simulink model "parallel_three_phase_converter"  (R2022b)
settings: Solver=VariableStepAuto  StartTime=0.0  StopTime=2  FixedStep=1e-6  MaxStep=1e-7  RelTol=1e-5
model workspace (MAT data in the model file):
  wr = 314.159265359
undefined symbols (not defined in the file): DiscIntNeverNeededParam, Ts
libraries: spsMosfetLib x12, spsCurrentMeasurementLib x7, dspsigops x7, slpidlib x5, simulink x3, spsThreePhaseSeriesRLCBranchLib x3, spsVoltageMeasurementLib x3, spsDCVoltageSourceLib x1, spsThreePhaseBreakerLib x1, spspowerguiLib x1
settings Model: Creator=SSC  LastModifiedBy=SSC

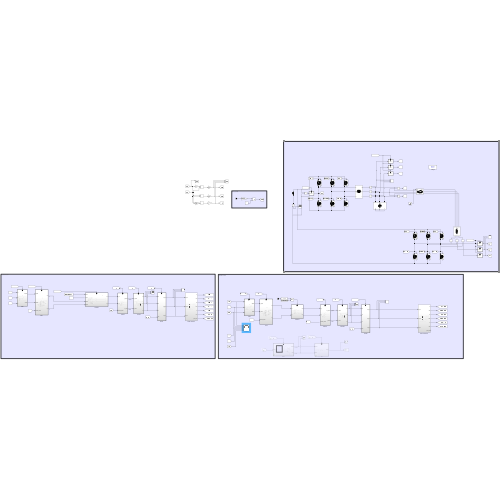
[thumbnail: Simulink's stored preview of the top-level diagram]
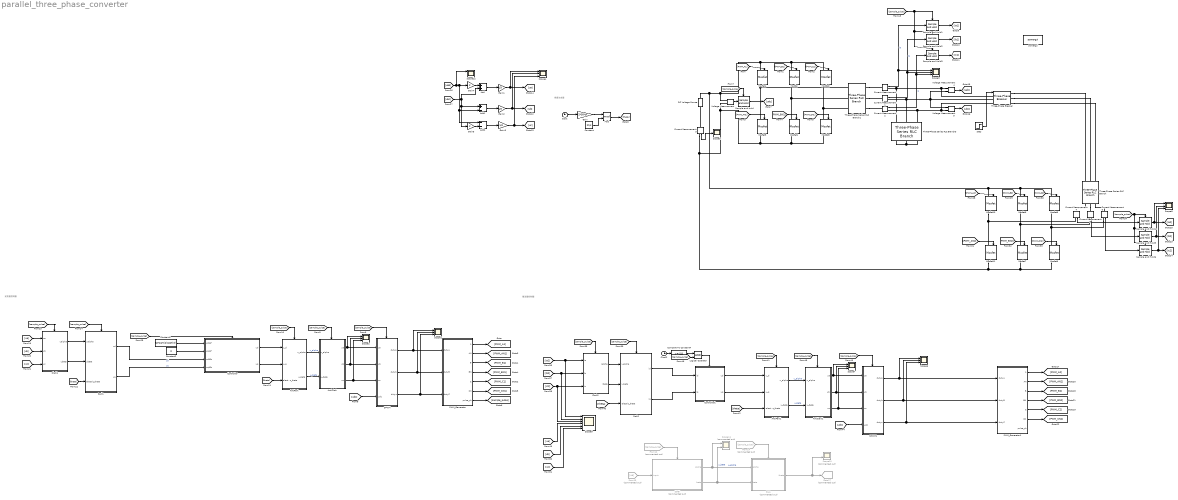
== system parallel_three_phase_converter ==
  note: 角度生成器
  note: 逆变器控制器
  note: 整流器控制器
  Add : Sum
  Add1 : Sum  Inputs=+-
  Add2 : Sum  Inputs=--
  AntiClark : Subsystem
  AntiClark1 : Subsystem
  AntiPark : Subsystem
  AntiPark1 : Subsystem
  Clark1 : Subsystem
  Clark2 : Subsystem
  Clock : Clock
  Clock2 : Clock
  Compare To Constant4 : simulink/Logic and Bit Operations/Compare To Constant  relop=>=  const=0.8  OutDataTypeStr=boolean
  Constant : Constant  Value=2*pi
  Constant1 : Constant  Value=32*sqrt(2)/sqrt(3)
  Constant2 : Constant  Value=0
  Controller : Subsystem
  Controller1 : Subsystem
  Current Measurement{,1..6} (7 alike) : spsCurrentMeasurementLib/Current Measurement  PhasorSimulation=off  OutputType=Complex  PSBequivalent=0
  DC Voltage Source : spsDCVoltageSourceLib/DC Voltage Source  Amplitude=56  Measurements=None
  From12 : From  Commented=on  GotoTag=sample_pulse
  From13 : From  Commented=on  GotoTag=ua
  From14 : From  Commented=on  GotoTag=sample_pulse
  Gain : Gain  Gain=2*50*pi
  Gain1 : Gain  Gain=1/3
  Gain2 : Gain  Gain=1/3
  Gain3 : Gain  Gain=1/3
  Gain4 : Gain  Gain=2
  Gain5 : Gain  Gain=2
  Goto27 : Goto  Commented=on  GotoTag=us_theta
  Logical Operator : Logic  AllPortsSameDT=off  OutDataTypeStr=boolean
  Mod : Math  Operator=mod
  Mosfet{,1..11} (12 alike) : spsMosfetLib/Mosfet  Ron=0.1  Lon=0  Rd=0.01  Vfd=0  IC=0  Rs=1e5  Cs=inf  Measurements=on
  PLL1 : Subsystem  Commented=on  TreatAsAtomicUnit=on
  PWM_Generator : Subsystem
  PWM_Generator1 : Subsystem
  Park1 : Subsystem
  Park2 : Subsystem
  SOGI : Subsystem  Commented=on  TreatAsAtomicUnit=on
  SPWM : Subsystem
  SPWM1 : Subsystem
  Sample and Hold{,1..6} (7 alike) : dspsigops/Sample and Hold  trig=Rising edge  initCond=0  latchinput=off
  Scope{1..4,6..8,12} (8 alike) : Scope  NumInputPorts=3
  Scope10 : Scope  Commented=on  NumInputPorts=2
  Scope11 : Scope  Commented=on  NumInputPorts=2
  Scope5 : Scope
  Scope9 : Scope  NumInputPorts=6
  Step : Step  Time=0.8  SampleTime=0
  Three-Phase Series RLC Branch : spsThreePhaseSeriesRLCBranchLib/Three-Phase Series RLC Branch  LConnTagsString=A|B|C  RConnTagsString=A|B|C  BranchType=L  Resistance=0  Inductance=2e-3  Capacitance=1e-6  Measurements=None
  Three-Phase Series RLC Branch1 : spsThreePhaseSeriesRLCBranchLib/Three-Phase Series RLC Branch  LConnTagsString=A|B|C  RConnTagsString=A|B|C  BranchType=L  Resistance=0  Inductance=2e-3  Capacitance=1e-6  Measurements=None
  Three-Phase Series RLC Branch3 : spsThreePhaseSeriesRLCBranchLib/Three-Phase Series RLC Branch  LConnTagsString=A|B|C  RConnTagsString=A|B|C  BranchType=C  Resistance=0  Inductance=10e-3  Capacitance=25e-6  Measurements=None
  Three-Phase Breaker : spsThreePhaseBreakerLib/Three-Phase Breaker  InitialState=open  SwitchA=on  SwitchB=on  SwitchC=on  SwitchTimes="[1/60  5/60]"  External=on  BreakerResistance=0.01  SnubberResistance=1e6  SnubberCapacitance=inf  Measurements=None
  Voltage Measurement : spsVoltageMeasurementLib/Voltage Measurement  PhasorSimulation=off  OutputType=Complex  PSBequivalent=0
  Voltage Measurement4 : spsVoltageMeasurementLib/Voltage Measurement  PhasorSimulation=off  OutputType=Complex  PSBequivalent=0
  Voltage Measurement5 : spsVoltageMeasurementLib/Voltage Measurement  PhasorSimulation=off  OutputType=Complex  PSBequivalent=0
  powergui : spspowerguiLib/powergui  Priority=1  SimulationMode=Discrete  SampleTime=1e-7  frequency=60  Iterations=50  frequencyindice=0  Pbase=100e6  ErrMax=1e-4  UnitsV=kV  UnitsW=MW  buscounter=0  FunctionMessages=off  echomessages=off  EnableUseOfTLC=off  CurrentSourceSwitches=off  DisableSnubberDevices=off  DisableRonSwitches=off  DisableVfSwitches=off  DisplayEquations=off  AutomaticDiscreteSolvers=off  SolverType=Tustin/Backward Euler (TBE)  Interpol=off  ExternalGateDelay=off  methode=off  Ts=100  x0status=blocks  SPID=on  SwTol=0  HookPort=off  NonlinearTolerance=1e-4  nMaxIteration=100  ContinueOnMaxIteration=off  RestoreLinks=warning  ResistiveCurrentMeasurement=off  Frange=[0:2:500]  Ylog=off  Xlog=on  ShowGrid=off  save=off  variable=ZData  structure=0  ZoomFFT=off  StartTime=0.0  cycles=1  DisplayStyle=1  fundamental=60  FreqAxis=off  MaxFrequency=1000  frequencyindicesteady=1  RmsSteady=1  display=off
  wires:
  Add/1 -> Gain1/1
  [uab] -> Scope12/1, Gain4/1, Add2/1, Add1/2
  Voltage Measurement5/1 -> [ubc]
  Add2/1 -> Gain3/1
  Voltage Measurement4/1 -> [uab]
  [ubc] -> Add/2, Gain5/1, Add1/1
  Gain3/1 -> Scope4/3, [uc]
  [ub] -> Clark1/2(ub)
  [theta] -> Park1/3(electric_theta)
  Park1/2(uq) -> Controller/4(uqfdb)  "uq"
  Clark1/2(ubeta) -> Park1/2(ubeta)
  [sample_pulse] -> Sample and Hold/Trigger
  Controller/2(uq) -> AntiPark/2(u_q)
  [sample_pulse] -> Park1/Trigger
  [PWM_A1] -> Mosfet4/1
  Constant2/1 -> Controller/2(uqref)
  Constant1/1 -> Controller/1(udref)
  Sample and Hold3/1 -> [ic1]
  [sample_pulse] -> Clark1/Trigger
  PWM_Generator/3(B) -> [PWM_B1]
  Sample and Hold1/1 -> [ia1]
  Current Measurement1/1 -> Scope3/2, Sample and Hold2/1  "ib"
  AntiClark/2(ub) -> SPWM/2(ub), Scope2/2
  SPWM/1(dutya) -> Scope1/1, PWM_Generator/1(dutyA)
  SPWM/2(dutyb) -> Scope1/2, PWM_Generator/2(dutyB)
  [sample_pulse] -> Controller/Trigger
  Sample and Hold/1 -> [udc]
  [ua] -> Clark1/1(ua)
  [udc] -> SPWM/4(udc)
  Controller/1(ud) -> AntiPark/1(u_d)
  [sample_pulse] -> AntiPark/Trigger
  Sample and Hold2/1 -> [ib1]
  Constant/1 -> Mod/2
  AntiClark/3(uc) -> SPWM/3(uc), Scope2/3
  Current Measurement2/1 -> Scope3/3, Sample and Hold3/1  "ic"
  [PWM_BN1] -> Mosfet1/1
  [PWM_B1] -> Mosfet/1
  PWM_Generator/6(CN) -> [PWM_CN1]
  Current Measurement/1 -> Scope3/1, Sample and Hold1/1  "ia"
  PWM_Generator/2(AN) -> [PWM_AN1]
  PWM_Generator/4(BN) -> [PWM_BN1]
  [sample_pulse] -> AntiClark/Trigger
  Voltage Measurement/1 -> Sample and Hold/1
  PWM_Generator/1(A) -> [PWM_A1]
  [PWM_AN1] -> Mosfet5/1
  [sample_pulse] -> SPWM/Trigger
  PWM_Generator/7(pulse_sh) -> [sample_pulse]
  SPWM/3(dutyc) -> Scope1/3, PWM_Generator/3(dutyC)
  [PWM_CN1] -> Mosfet3/1
  Clock/1 -> Gain/1
  [uc] -> Clark1/3(uc)
  AntiClark/1(ua) -> SPWM/1(ua), Scope2/1
  Gain5/1 -> Add2/2
  Gain/1 -> Mod/1
  Gain4/1 -> Add/1
  PWM_Generator/5(C) -> [PWM_C1]
  [PWM_C1] -> Mosfet2/1
  Gain2/1 -> Scope4/2, [ub]
  Mod/1 -> [theta]
  [theta] -> AntiPark/3(electric_theta)
  Add1/1 -> Gain2/1
  [sample_pulse] -> Sample and Hold1/Trigger, Sample and Hold3/Trigger, Sample and Hold2/Trigger
  [PWM_C2] -> Mosfet8/1
  [PWM_CN2] -> Mosfet9/1
  [PWM_AN2] -> Mosfet11/1
  [PWM_BN2] -> Mosfet7/1
  [PWM_B2] -> Mosfet6/1
  [PWM_A2] -> Mosfet10/1
  SPWM1/1(dutya) -> PWM_Generator1/1(dutyA), Scope6/1
  SPWM1/2(dutyb) -> PWM_Generator1/2(dutyB), Scope6/2
  SPWM1/3(dutyc) -> PWM_Generator1/3(dutyC), Scope6/3
  Current Measurement3/1 -> Scope5/1
  Current Measurement5/1 -> Sample and Hold5/1
  Current Measurement4/1 -> Sample and Hold4/1
  Current Measurement6/1 -> Sample and Hold6/1
  [sample_pulse] -> Sample and Hold4/Trigger, Sample and Hold6/Trigger, Sample and Hold5/Trigger
  Clark2/2(ibeta) -> Park2/2(i_beta)
  [sample_pulse] -> Park2/Trigger
  [ib2] -> Scope9/2, Clark2/2(ib)
  [ia2] -> Scope9/1, Clark2/1(ia)
  [sample_pulse] -> Clark2/Trigger
  Clark2/1(ialpha) -> Park2/1(i_alpha)
  AntiClark1/1(ua) -> SPWM1/1(ua), Scope7/1
  [sample_pulse] -> AntiClark1/Trigger
  [sample_pulse] -> SPWM1/Trigger
  AntiPark1/1(u_alpha) -> AntiClark1/1(u_alpha)  "u_alpha"
  [sample_pulse] -> AntiPark1/Trigger
  AntiClark1/3(uc) -> SPWM1/3(uc), Scope7/3
  [udc] -> SPWM1/4(udc)
  AntiClark1/2(ub) -> SPWM1/2(ub), Scope7/2
  AntiPark1/2(u_beta) -> AntiClark1/2(u_beta)  "u_beta"
  Park2/1(id) -> Controller1/1(id)
  Park2/2(iq) -> Controller1/2(iq)
  PWM_Generator1/1(A) -> [PWM_A2]
  PWM_Generator1/2(AN) -> [PWM_AN2]
  PWM_Generator1/4(BN) -> [PWM_BN2]
  PWM_Generator1/3(B) -> [PWM_B2]
  PWM_Generator1/5(C) -> [PWM_C2]
  PWM_Generator1/6(CN) -> [PWM_CN2]
  Controller1/1(ud) -> AntiPark1/1(u_d)
  Controller1/2(uq) -> AntiPark1/2(u_q)
  AntiPark/1(u_alpha) -> AntiClark/1(u_alpha)  "u_alpha"
  AntiPark/2(u_beta) -> AntiClark/2(u_beta)  "u_beta"
  Gain1/1 -> Scope4/1, [ua]
  Clark1/1(ualpha) -> Park1/1(ualpha)
  [theta] -> AntiPark1/3(electric_theta)
  Park1/1(ud) -> Controller/3(udfdb)  "ud"
  [ua] -> Scope9/4
  [uc] -> Scope9/6
  Sample and Hold4/1 -> Scope8/1, [ia2]
  Sample and Hold5/1 -> Scope8/2, [ib2]
  Sample and Hold6/1 -> Scope8/3, [ic2]
  [theta] -> Park2/3(electric_theta)
  [ub] -> Scope9/5
  Clock2/1 -> Compare To Constant4/1
  Compare To Constant4/1 -> Logical Operator/1
  [sample_pulse] -> Logical Operator/2
  Logical Operator/1 -> Controller1/Trigger
  [ic2] -> Scope9/3, Clark2/3(ic)
  SOGI/1(alpha) -> PLL1/1(alpha), Scope11/1  "u_alpha"
  From12/1 -> SOGI/Trigger
  SOGI/2(beta) -> PLL1/2(beta), Scope11/2  "u_beta"
  From13/1 -> SOGI/1(input)
  From14/1 -> PLL1/Trigger
  PLL1/1(theta) -> Scope10/2, Goto27/1
  Step/1 -> Three-Phase Breaker/1
  connections:
  Mosfet11/RConn1 -- Mosfet1/RConn1 -- Mosfet3/RConn1 -- Mosfet5/RConn1 -- Voltage Measurement/LConn2 -- Current Measurement3/RConn1 -- Mosfet9/RConn1 -- Mosfet7/RConn1
  Mosfet8/LConn1 -- Mosfet6/LConn1 -- Mosfet4/LConn1 -- Mosfet/LConn1 -- Mosfet2/LConn1 -- Voltage Measurement/LConn1 -- DC Voltage Source/RConn1 -- Mosfet10/LConn1
  Mosfet/RConn1 -- Three-Phase Series RLC Branch1/LConn2 -- Mosfet1/LConn1
  Mosfet4/RConn1 -- Three-Phase Series RLC Branch1/LConn1 -- Mosfet5/LConn1
  Mosfet2/RConn1 -- Three-Phase Series RLC Branch1/LConn3 -- Mosfet3/LConn1
  Three-Phase Series RLC Branch1/RConn1 -- Current Measurement/LConn1
  Three-Phase Series RLC Branch1/RConn2 -- Current Measurement1/LConn1
  Three-Phase Series RLC Branch1/RConn3 -- Current Measurement2/LConn1
  Mosfet9/LConn1 -- Current Measurement6/RConn1 -- Mosfet8/RConn1
  Mosfet10/RConn1 -- Current Measurement4/RConn1 -- Mosfet11/LConn1
  Mosfet7/LConn1 -- Current Measurement5/RConn1 -- Mosfet6/RConn1
  Current Measurement/RConn1 -- Three-Phase Breaker/LConn1 -- Voltage Measurement4/LConn1 -- Three-Phase Series RLC Branch3/LConn1
  Current Measurement1/RConn1 -- Three-Phase Breaker/LConn2 -- Voltage Measurement5/LConn1 -- Voltage Measurement4/LConn2 -- Three-Phase Series RLC Branch3/LConn2
  Current Measurement2/RConn1 -- Three-Phase Breaker/LConn3 -- Voltage Measurement5/LConn2 -- Three-Phase Series RLC Branch3/LConn3
  Three-Phase Series RLC Branch/RConn1 -- Current Measurement4/LConn1
  Three-Phase Series RLC Branch/RConn2 -- Current Measurement5/LConn1
  Three-Phase Series RLC Branch/RConn3 -- Current Measurement6/LConn1
  Current Measurement3/LConn1 -- DC Voltage Source/LConn1
  Three-Phase Series RLC Branch3/RConn1 -- Three-Phase Series RLC Branch3/RConn3 -- Three-Phase Series RLC Branch3/RConn2
  Three-Phase Breaker/RConn3 -- Three-Phase Series RLC Branch/LConn3
  Three-Phase Breaker/RConn2 -- Three-Phase Series RLC Branch/LConn2
  Three-Phase Breaker/RConn1 -- Three-Phase Series RLC Branch/LConn1

== system parallel_three_phase_converter/AntiClark ==
  u_alpha : Inport
  u_beta : Inport  Port=2
  Trigger : TriggerPort  VariantControl=(inherit)
  Gain : Gain  Gain=-1/2
  Gain1 : Gain  Gain=sqrt(3)/2
  Sum : Sum  Inputs=|++
  Sum1 : Sum  Inputs=-+|
  ua : Outport
  ub : Outport  Port=2
  uc : Outport  Port=3
  wires:
  Sum1/1 -> uc/1
  Gain1/1 -> Sum1/1, Sum/2
  Sum/1 -> ub/1
  Gain/1 -> Sum/1, Sum1/2
  u_beta/1 -> Gain1/1
  u_alpha/1 -> ua/1, Gain/1

== system parallel_three_phase_converter/AntiClark1 ==
  u_alpha : Inport
  u_beta : Inport  Port=2
  Trigger : TriggerPort  VariantControl=(inherit)
  Gain : Gain  Gain=-1/2
  Gain1 : Gain  Gain=sqrt(3)/2
  Sum : Sum  Inputs=|++
  Sum1 : Sum  Inputs=-+|
  ua : Outport
  ub : Outport  Port=2
  uc : Outport  Port=3
  wires:
  Sum1/1 -> uc/1
  Gain1/1 -> Sum1/1, Sum/2
  Sum/1 -> ub/1
  Gain/1 -> Sum/1, Sum1/2
  u_beta/1 -> Gain1/1
  u_alpha/1 -> ua/1, Gain/1

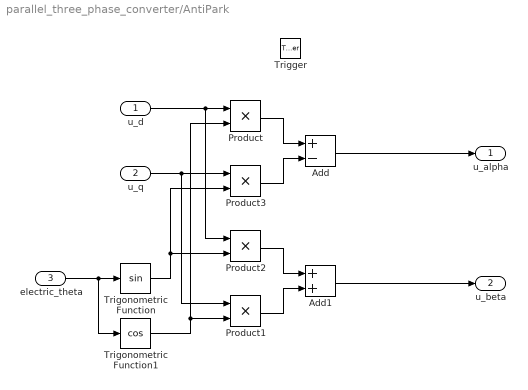
== system parallel_three_phase_converter/AntiPark ==
  u_d : Inport
  u_q : Inport  Port=2
  electric_theta : Inport  Port=3
  Trigger : TriggerPort  VariantControl=(inherit)
  Add : Sum  Inputs=+-
  Add1 : Sum
  Product{,1..3} (4 alike) : Product
  Trigonometric Function : Trigonometry
  Trigonometric Function1 : Trigonometry  Operator=cos
  u_alpha : Outport
  u_beta : Outport  Port=2
  wires:
  electric_theta/1 -> Trigonometric Function1/1, Trigonometric Function/1
  u_d/1 -> Product2/1, Product/1
  Trigonometric Function1/1 -> Product/2, Product1/2
  u_q/1 -> Product1/1, Product3/1
  Trigonometric Function/1 -> Product2/2, Product3/2
  Product/1 -> Add/1
  Product3/1 -> Add/2
  Add/1 -> u_alpha/1
  Product2/1 -> Add1/1
  Product1/1 -> Add1/2
  Add1/1 -> u_beta/1

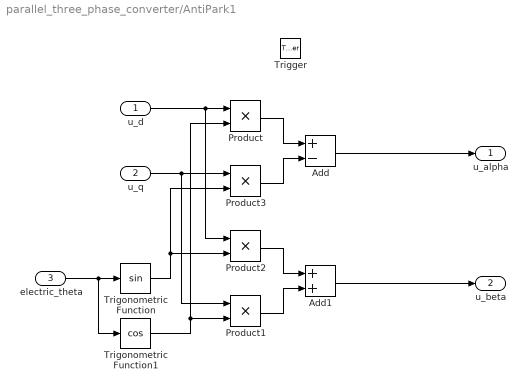
== system parallel_three_phase_converter/AntiPark1 ==
  u_d : Inport
  u_q : Inport  Port=2
  electric_theta : Inport  Port=3
  Trigger : TriggerPort  VariantControl=(inherit)
  Add : Sum  Inputs=+-
  Add1 : Sum
  Product{,1..3} (4 alike) : Product
  Trigonometric Function : Trigonometry
  Trigonometric Function1 : Trigonometry  Operator=cos
  u_alpha : Outport
  u_beta : Outport  Port=2
  wires:
  electric_theta/1 -> Trigonometric Function1/1, Trigonometric Function/1
  u_d/1 -> Product2/1, Product/1
  Trigonometric Function1/1 -> Product/2, Product1/2
  u_q/1 -> Product1/1, Product3/1
  Trigonometric Function/1 -> Product2/2, Product3/2
  Product/1 -> Add/1
  Product3/1 -> Add/2
  Add/1 -> u_alpha/1
  Product2/1 -> Add1/1
  Product1/1 -> Add1/2
  Add1/1 -> u_beta/1

== system parallel_three_phase_converter/Clark1 ==
  ua : Inport
  ub : Inport  Port=2
  uc : Inport  Port=3
  Trigger : TriggerPort  VariantControl=(inherit)
  Add : Sum
  Add1 : Sum  Inputs=+-
  Add2 : Sum  Inputs=+-
  Gain : Gain  Gain=2/3
  Gain1 : Gain  Gain=1/3
  Gain2 : Gain  Gain=sqrt(3)/3
  ualpha : Outport
  ubeta : Outport  Port=2
  wires:
  ua/1 -> Gain/1
  ub/1 -> Add1/1, Add/1
  uc/1 -> Add/2, Add1/2
  Add/1 -> Gain1/1
  Add1/1 -> Gain2/1
  Gain/1 -> Add2/1
  Gain1/1 -> Add2/2
  Add2/1 -> ualpha/1
  Gain2/1 -> ubeta/1

== system parallel_three_phase_converter/Clark2 ==
  ia : Inport
  ib : Inport  Port=2
  ic : Inport  Port=3
  Trigger : TriggerPort  VariantControl=(inherit)
  Add : Sum
  Add1 : Sum  Inputs=+-
  Add2 : Sum  Inputs=+-
  Gain : Gain  Gain=2/3
  Gain1 : Gain  Gain=1/3
  Gain2 : Gain  Gain=sqrt(3)/3
  ialpha : Outport
  ibeta : Outport  Port=2
  wires:
  ia/1 -> Gain/1
  ib/1 -> Add1/1, Add/1
  ic/1 -> Add/2, Add1/2
  Add/1 -> Gain1/1
  Add1/1 -> Gain2/1
  Gain/1 -> Add2/1
  Gain1/1 -> Add2/2
  Add2/1 -> ialpha/1
  Gain2/1 -> ibeta/1

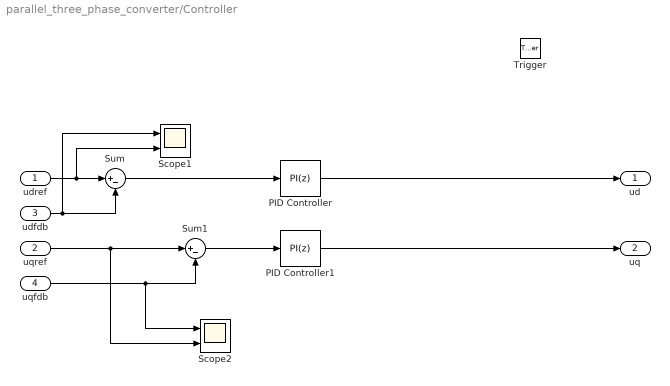
== system parallel_three_phase_converter/Controller ==
  udref : Inport
  uqref : Inport  Port=2
  udfdb : Inport  Port=3
  uqfdb : Inport  Port=4
  Trigger : TriggerPort  VariantControl=(inherit)
  PID Controller : slpidlib/PID Controller  Controller=PI  Form=Parallel  TimeDomain=Discrete-time  UseExternalTs=off  SampleTime=-1  IntegratorMethod=Forward Euler  FilterMethod=Forward Euler  ControllerParametersSource=internal  P=0.01  I=5  UseKiTs=off  D=0  N=100  UseFilter=on  TunerSelectOption=Transfer Function Based (PID Tuner App)  InitialConditionSource=internal  InitialConditionForIntegrator=0  InitialConditionForFilter=0  DifferentiatorICPrevScaledInput=0  ExternalReset=none  TrackingMode=off  Kt=1  LimitOutput=on  SatLimitsSource=internal  UpperSaturationLimit=60/2  LowerSaturationLimit=-60/2  LinearizeAsGain=on  AntiWindupMode=clamping  Kb=1  LimitIntegrator=off  UpperIntegratorSaturationLimit=inf  LowerIntegratorSaturationLimit=-inf  POutMin=[]  POutMax=[]  IOutMin=[]  IOutMax=[]  DOutMin=[]  DOutMax=[]  NOutMin=[]  NOutMax=[]  SumOutMin=[]  SumOutMax=[]  SaturationOutMin=[]  SaturationOutMax=[]  PParamMin=[]  PParamMax=[]  IParamMin=[]  IParamMax=[]  DParamMin=[]  DParamMax=[]  NParamMin=[]  NParamMax=[]  KbParamMin=[]  KbParamMax=[]  KtParamMin=[]  KtParamMax=[]  KbOutMin=[]  KbOutMax=[]  KtOutMin=[]  KtOutMax=[]  IntegratorOutMin=[]  IntegratorOutMax=[]  FilterOutMin=[]  FilterOutMax=[]  SumI1OutMin=[]  SumI1OutMax=[]  SumI2OutMin=[]  SumI2OutMax=[]  SumI3OutMin=[]  SumI3OutMax=[]  SumI4OutMin=[]  SumI4OutMax=[]  SumDOutMin=[]  SumDOutMax=[]  DifferentiatorOutMin=[]  DifferentiatorOutMax=[]  FilterDiffOutCoefMin=[]  FilterDiffOutCoefMax=[]  ReciprocalOutMin=[]  ReciprocalOutMax=[]  SumDenOutMin=[]  SumDenOutMax=[]  SumNumOutMin=[]  SumNumOutMax=[]  DivideOutMin=[]  DivideOutMax=[]  UdiffTsProdOutMin=[]  UdiffTsProdOutMax=[]  NTsProdOutMin=[]  NTsProdOutMax=[]  UintegralTsProdOutMin=[]  UintegralTsProdOutMax=[]  UngainTsProdOutMin=[]  UngainTsProdOutMax=[]  ClampingZeroOutDataTypeStr=Inherit: Inherit via back propagation  ClampingZeroOutMin=[]  ClampingZeroOutMax=[]  FilterDenConstantOutDataTypeStr=Inherit: Inherit via back propagation  FilterDenConstantOutMin=[]  FilterDenConstantOutMax=[]  PCopyOutDataTypeStr=Inherit: Inherit via back propagation  PCopyOutMin=[]  PCopyOutMax=[]  NCopyOutDataTypeStr=Inherit: Inherit via back propagation  NCopyOutMin=[]  NCopyOutMax=[]  IntegratorContinuousStateAttributes=''  IntegratorStateMustResolveToSignalObject=off  IntegratorRTWStateStorageClass=Auto  FilterContinuousStateAttributes=''  FilterStateMustResolveToSignalObject=off  FilterRTWStateStorageClass=Auto  ParallelPVariant=InternalParameters  IdealPVariant=Disabled  IVariant=InternalParameters  DVariant=Disabled  IntegratorVariant=Discrete  SatVariant=Enabled  AWVariant=DiscClampingParallel  PCopyVariant=Disabled  TRVariant=Disabled  FdbkBlocksVariant=Forward  IdealPFdbkVariant=Disabled  SatFdbkVariant=Disabled  DerivativeFilterVariant=Disabled  NVariant=Disabled  NCopyVariant=Disabled_SignalSpec  FilterICVariant=Disabled  IntegratorICVariant=InternalICs  ExternalResetVariant=Disabled  TRSumVariant=Passthrough  SumFdbkVariant=Disabled  SumVariant=Sum_PI  TsampFilterVariant=InternalTs  TsampNgainVariant=Passthrough  TsampIntegralVariant=Passthrough  ExternalSaturationOutDataTypeStr=Inherit: Same as second input
  PID Controller1 : slpidlib/PID Controller  Controller=PI  Form=Parallel  TimeDomain=Discrete-time  UseExternalTs=off  SampleTime=-1  IntegratorMethod=Forward Euler  FilterMethod=Forward Euler  ControllerParametersSource=internal  P=0.01  I=5  UseKiTs=off  D=0  N=100  UseFilter=on  TunerSelectOption=Transfer Function Based (PID Tuner App)  InitialConditionSource=internal  InitialConditionForIntegrator=0  InitialConditionForFilter=0  DifferentiatorICPrevScaledInput=0  ExternalReset=none  TrackingMode=off  Kt=1  LimitOutput=on  SatLimitsSource=internal  UpperSaturationLimit=60/2  LowerSaturationLimit=-60/2  LinearizeAsGain=on  AntiWindupMode=clamping  Kb=1  LimitIntegrator=off  UpperIntegratorSaturationLimit=inf  LowerIntegratorSaturationLimit=-inf  POutMin=[]  POutMax=[]  IOutMin=[]  IOutMax=[]  DOutMin=[]  DOutMax=[]  NOutMin=[]  NOutMax=[]  SumOutMin=[]  SumOutMax=[]  SaturationOutMin=[]  SaturationOutMax=[]  PParamMin=[]  PParamMax=[]  IParamMin=[]  IParamMax=[]  DParamMin=[]  DParamMax=[]  NParamMin=[]  NParamMax=[]  KbParamMin=[]  KbParamMax=[]  KtParamMin=[]  KtParamMax=[]  KbOutMin=[]  KbOutMax=[]  KtOutMin=[]  KtOutMax=[]  IntegratorOutMin=[]  IntegratorOutMax=[]  FilterOutMin=[]  FilterOutMax=[]  SumI1OutMin=[]  SumI1OutMax=[]  SumI2OutMin=[]  SumI2OutMax=[]  SumI3OutMin=[]  SumI3OutMax=[]  SumI4OutMin=[]  SumI4OutMax=[]  SumDOutMin=[]  SumDOutMax=[]  DifferentiatorOutMin=[]  DifferentiatorOutMax=[]  FilterDiffOutCoefMin=[]  FilterDiffOutCoefMax=[]  ReciprocalOutMin=[]  ReciprocalOutMax=[]  SumDenOutMin=[]  SumDenOutMax=[]  SumNumOutMin=[]  SumNumOutMax=[]  DivideOutMin=[]  DivideOutMax=[]  UdiffTsProdOutMin=[]  UdiffTsProdOutMax=[]  NTsProdOutMin=[]  NTsProdOutMax=[]  UintegralTsProdOutMin=[]  UintegralTsProdOutMax=[]  UngainTsProdOutMin=[]  UngainTsProdOutMax=[]  ClampingZeroOutDataTypeStr=Inherit: Inherit via back propagation  ClampingZeroOutMin=[]  ClampingZeroOutMax=[]  FilterDenConstantOutDataTypeStr=Inherit: Inherit via back propagation  FilterDenConstantOutMin=[]  FilterDenConstantOutMax=[]  PCopyOutDataTypeStr=Inherit: Inherit via back propagation  PCopyOutMin=[]  PCopyOutMax=[]  NCopyOutDataTypeStr=Inherit: Inherit via back propagation  NCopyOutMin=[]  NCopyOutMax=[]  IntegratorContinuousStateAttributes=''  IntegratorStateMustResolveToSignalObject=off  IntegratorRTWStateStorageClass=Auto  FilterContinuousStateAttributes=''  FilterStateMustResolveToSignalObject=off  FilterRTWStateStorageClass=Auto  ParallelPVariant=InternalParameters  IdealPVariant=Disabled  IVariant=InternalParameters  DVariant=Disabled  IntegratorVariant=Discrete  SatVariant=Enabled  AWVariant=DiscClampingParallel  PCopyVariant=Disabled  TRVariant=Disabled  FdbkBlocksVariant=Forward  IdealPFdbkVariant=Disabled  SatFdbkVariant=Disabled  DerivativeFilterVariant=Disabled  NVariant=Disabled  NCopyVariant=Disabled_SignalSpec  FilterICVariant=Disabled  IntegratorICVariant=InternalICs  ExternalResetVariant=Disabled  TRSumVariant=Passthrough  SumFdbkVariant=Disabled  SumVariant=Sum_PI  TsampFilterVariant=InternalTs  TsampNgainVariant=Passthrough  TsampIntegralVariant=Passthrough  ExternalSaturationOutDataTypeStr=Inherit: Same as second input
  Scope1 : Scope  NumInputPorts=2
  Scope2 : Scope  NumInputPorts=2
  Sum : Sum  Inputs=|+-
  Sum1 : Sum  Inputs=|+-
  ud : Outport
  uq : Outport  Port=2
  wires:
  PID Controller1/1 -> uq/1
  uqref/1 -> Scope2/2, Sum1/1
  PID Controller/1 -> ud/1
  udref/1 -> Scope1/2, Sum/1
  Sum/1 -> PID Controller/1
  Sum1/1 -> PID Controller1/1
  udfdb/1 -> Sum/2, Scope1/1
  uqfdb/1 -> Scope2/1, Sum1/2

== system parallel_three_phase_converter/Controller1 ==
  id : Inport
  iq : Inport  Port=2
  Trigger : TriggerPort  VariantControl=(inherit)
  Constant10 : Constant  Value=0
  Constant9 : Constant  Value=0.5
  PID Controller1 : slpidlib/PID Controller  Controller=PI  Form=Parallel  TimeDomain=Discrete-time  UseExternalTs=off  SampleTime=-1  IntegratorMethod=Forward Euler  FilterMethod=Forward Euler  ControllerParametersSource=internal  P=10  I=100  UseKiTs=off  D=0  N=100  UseFilter=on  TunerSelectOption=Transfer Function Based (PID Tuner App)  InitialConditionSource=internal  InitialConditionForIntegrator=0  InitialConditionForFilter=0  DifferentiatorICPrevScaledInput=0  ExternalReset=none  TrackingMode=off  Kt=1  LimitOutput=on  SatLimitsSource=internal  UpperSaturationLimit=60/2  LowerSaturationLimit=-60/2  LinearizeAsGain=on  AntiWindupMode=none  Kb=1  LimitIntegrator=off  UpperIntegratorSaturationLimit=inf  LowerIntegratorSaturationLimit=-inf  POutMin=[]  POutMax=[]  IOutMin=[]  IOutMax=[]  DOutMin=[]  DOutMax=[]  NOutMin=[]  NOutMax=[]  SumOutMin=[]  SumOutMax=[]  SaturationOutMin=[]  SaturationOutMax=[]  PParamMin=[]  PParamMax=[]  IParamMin=[]  IParamMax=[]  DParamMin=[]  DParamMax=[]  NParamMin=[]  NParamMax=[]  KbParamMin=[]  KbParamMax=[]  KtParamMin=[]  KtParamMax=[]  KbOutMin=[]  KbOutMax=[]  KtOutMin=[]  KtOutMax=[]  IntegratorOutMin=[]  IntegratorOutMax=[]  FilterOutMin=[]  FilterOutMax=[]  SumI1OutMin=[]  SumI1OutMax=[]  SumI2OutMin=[]  SumI2OutMax=[]  SumI3OutMin=[]  SumI3OutMax=[]  SumI4OutMin=[]  SumI4OutMax=[]  SumDOutMin=[]  SumDOutMax=[]  DifferentiatorOutMin=[]  DifferentiatorOutMax=[]  FilterDiffOutCoefMin=[]  FilterDiffOutCoefMax=[]  ReciprocalOutMin=[]  ReciprocalOutMax=[]  SumDenOutMin=[]  SumDenOutMax=[]  SumNumOutMin=[]  SumNumOutMax=[]  DivideOutMin=[]  DivideOutMax=[]  UdiffTsProdOutMin=[]  UdiffTsProdOutMax=[]  NTsProdOutMin=[]  NTsProdOutMax=[]  UintegralTsProdOutMin=[]  UintegralTsProdOutMax=[]  UngainTsProdOutMin=[]  UngainTsProdOutMax=[]  ClampingZeroOutDataTypeStr=Inherit: Inherit via back propagation  ClampingZeroOutMin=[]  ClampingZeroOutMax=[]  FilterDenConstantOutDataTypeStr=Inherit: Inherit via back propagation  FilterDenConstantOutMin=[]  FilterDenConstantOutMax=[]  PCopyOutDataTypeStr=Inherit: Inherit via back propagation  PCopyOutMin=[]  PCopyOutMax=[]  NCopyOutDataTypeStr=Inherit: Inherit via back propagation  NCopyOutMin=[]  NCopyOutMax=[]  IntegratorContinuousStateAttributes=''  IntegratorStateMustResolveToSignalObject=off  IntegratorRTWStateStorageClass=Auto  FilterContinuousStateAttributes=''  FilterStateMustResolveToSignalObject=off  FilterRTWStateStorageClass=Auto  ParallelPVariant=InternalParameters  IdealPVariant=Disabled  IVariant=InternalParameters  DVariant=Disabled  IntegratorVariant=Discrete  SatVariant=Enabled  AWVariant=Passthrough  PCopyVariant=Disabled  TRVariant=Disabled  FdbkBlocksVariant=Forward  IdealPFdbkVariant=Disabled  SatFdbkVariant=Disabled  DerivativeFilterVariant=Disabled  NVariant=Disabled  NCopyVariant=Disabled_SignalSpec  FilterICVariant=Disabled  IntegratorICVariant=InternalICs  ExternalResetVariant=Disabled  TRSumVariant=Passthrough  SumFdbkVariant=Disabled  SumVariant=Sum_PI  TsampFilterVariant=InternalTs  TsampNgainVariant=Passthrough  TsampIntegralVariant=Passthrough  ExternalSaturationOutDataTypeStr=Inherit: Same as second input
  PID Controller2 : slpidlib/PID Controller  Controller=PI  Form=Parallel  TimeDomain=Discrete-time  UseExternalTs=off  SampleTime=-1  IntegratorMethod=Forward Euler  FilterMethod=Forward Euler  ControllerParametersSource=internal  P=10  I=100  UseKiTs=off  D=0  N=100  UseFilter=on  TunerSelectOption=Transfer Function Based (PID Tuner App)  InitialConditionSource=internal  InitialConditionForIntegrator=0  InitialConditionForFilter=0  DifferentiatorICPrevScaledInput=0  ExternalReset=none  TrackingMode=off  Kt=1  LimitOutput=on  SatLimitsSource=internal  UpperSaturationLimit=60/2  LowerSaturationLimit=-60/2  LinearizeAsGain=on  AntiWindupMode=none  Kb=1  LimitIntegrator=off  UpperIntegratorSaturationLimit=inf  LowerIntegratorSaturationLimit=-inf  POutMin=[]  POutMax=[]  IOutMin=[]  IOutMax=[]  DOutMin=[]  DOutMax=[]  NOutMin=[]  NOutMax=[]  SumOutMin=[]  SumOutMax=[]  SaturationOutMin=[]  SaturationOutMax=[]  PParamMin=[]  PParamMax=[]  IParamMin=[]  IParamMax=[]  DParamMin=[]  DParamMax=[]  NParamMin=[]  NParamMax=[]  KbParamMin=[]  KbParamMax=[]  KtParamMin=[]  KtParamMax=[]  KbOutMin=[]  KbOutMax=[]  KtOutMin=[]  KtOutMax=[]  IntegratorOutMin=[]  IntegratorOutMax=[]  FilterOutMin=[]  FilterOutMax=[]  SumI1OutMin=[]  SumI1OutMax=[]  SumI2OutMin=[]  SumI2OutMax=[]  SumI3OutMin=[]  SumI3OutMax=[]  SumI4OutMin=[]  SumI4OutMax=[]  SumDOutMin=[]  SumDOutMax=[]  DifferentiatorOutMin=[]  DifferentiatorOutMax=[]  FilterDiffOutCoefMin=[]  FilterDiffOutCoefMax=[]  ReciprocalOutMin=[]  ReciprocalOutMax=[]  SumDenOutMin=[]  SumDenOutMax=[]  SumNumOutMin=[]  SumNumOutMax=[]  DivideOutMin=[]  DivideOutMax=[]  UdiffTsProdOutMin=[]  UdiffTsProdOutMax=[]  NTsProdOutMin=[]  NTsProdOutMax=[]  UintegralTsProdOutMin=[]  UintegralTsProdOutMax=[]  UngainTsProdOutMin=[]  UngainTsProdOutMax=[]  ClampingZeroOutDataTypeStr=Inherit: Inherit via back propagation  ClampingZeroOutMin=[]  ClampingZeroOutMax=[]  FilterDenConstantOutDataTypeStr=Inherit: Inherit via back propagation  FilterDenConstantOutMin=[]  FilterDenConstantOutMax=[]  PCopyOutDataTypeStr=Inherit: Inherit via back propagation  PCopyOutMin=[]  PCopyOutMax=[]  NCopyOutDataTypeStr=Inherit: Inherit via back propagation  NCopyOutMin=[]  NCopyOutMax=[]  IntegratorContinuousStateAttributes=''  IntegratorStateMustResolveToSignalObject=off  IntegratorRTWStateStorageClass=Auto  FilterContinuousStateAttributes=''  FilterStateMustResolveToSignalObject=off  FilterRTWStateStorageClass=Auto  ParallelPVariant=InternalParameters  IdealPVariant=Disabled  IVariant=InternalParameters  DVariant=Disabled  IntegratorVariant=Discrete  SatVariant=Enabled  AWVariant=Passthrough  PCopyVariant=Disabled  TRVariant=Disabled  FdbkBlocksVariant=Forward  IdealPFdbkVariant=Disabled  SatFdbkVariant=Disabled  DerivativeFilterVariant=Disabled  NVariant=Disabled  NCopyVariant=Disabled_SignalSpec  FilterICVariant=Disabled  IntegratorICVariant=InternalICs  ExternalResetVariant=Disabled  TRSumVariant=Passthrough  SumFdbkVariant=Disabled  SumVariant=Sum_PI  TsampFilterVariant=InternalTs  TsampNgainVariant=Passthrough  TsampIntegralVariant=Passthrough  ExternalSaturationOutDataTypeStr=Inherit: Same as second input
  Scope1 : Scope  NumInputPorts=2
  Scope6 : Scope  NumInputPorts=2
  Sum2 : Sum  Inputs=|-+
  Sum3 : Sum  Inputs=|-+
  ud : Outport
  uq : Outport  Port=2
  wires:
  PID Controller2/1 -> ud/1
  id/1 -> Scope6/2, Sum2/2
  PID Controller1/1 -> uq/1
  Sum3/1 -> PID Controller1/1
  iq/1 -> Scope1/2, Sum3/2
  Sum2/1 -> PID Controller2/1
  Constant10/1 -> Scope1/1, Sum3/1
  Constant9/1 -> Scope6/1, Sum2/1

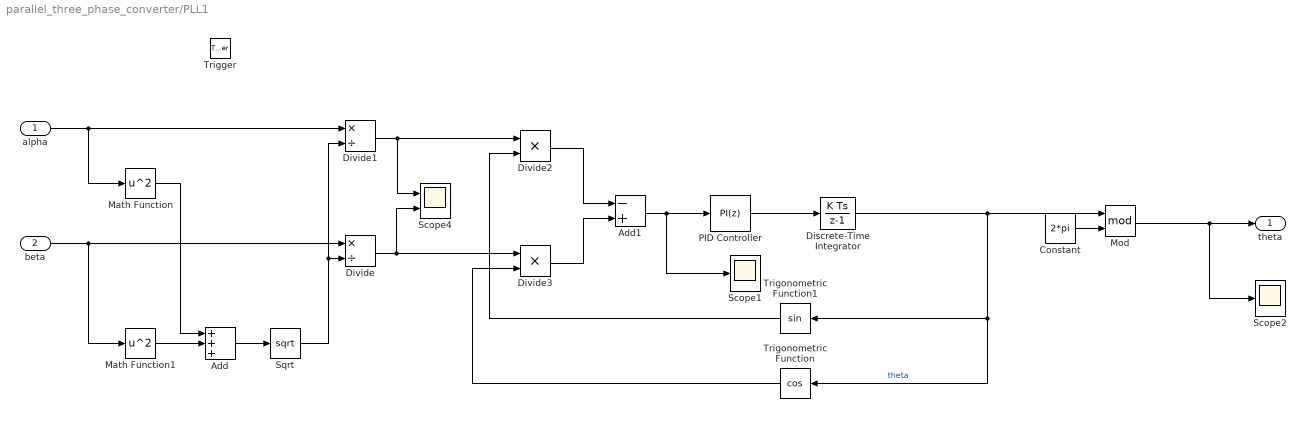
== system parallel_three_phase_converter/PLL1 ==
  alpha : Inport
  beta : Inport  Port=2
  Trigger : TriggerPort  VariantControl=(inherit)
  Add : Sum  Inputs=+++
  Add1 : Sum  Inputs=-+
  Constant : Constant  Value=2*pi
  Discrete-Time Integrator : DiscreteIntegrator  SampleTime=-1  ICPrevOutput=DiscIntNeverNeededParam  ICPrevScaledInput=DiscIntNeverNeededParam
  Divide : Product  Inputs=*/
  Divide1 : Product  Inputs=*/
  Divide2 : Product  Inputs=**
  Divide3 : Product  Inputs=**
  Math Function : Math  Operator=square
  Math Function1 : Math  Operator=square
  Mod : Math  Operator=mod
  PID Controller : slpidlib/PID Controller  Controller=PI  Form=Parallel  TimeDomain=Discrete-time  UseExternalTs=off  SampleTime=-1  IntegratorMethod=Forward Euler  FilterMethod=Forward Euler  ControllerParametersSource=internal  P=500  I=2000  UseKiTs=off  D=0  N=100  UseFilter=on  TunerSelectOption=Transfer Function Based (PID Tuner App)  InitialConditionSource=internal  InitialConditionForIntegrator=0  InitialConditionForFilter=0  DifferentiatorICPrevScaledInput=0  ExternalReset=none  TrackingMode=off  Kt=1  LimitOutput=off  SatLimitsSource=internal  UpperSaturationLimit=inf  LowerSaturationLimit=-inf  LinearizeAsGain=on  AntiWindupMode=none  Kb=1  LimitIntegrator=off  UpperIntegratorSaturationLimit=inf  LowerIntegratorSaturationLimit=-inf  POutMin=[]  POutMax=[]  IOutMin=[]  IOutMax=[]  DOutMin=[]  DOutMax=[]  NOutMin=[]  NOutMax=[]  SumOutMin=[]  SumOutMax=[]  SaturationOutMin=[]  SaturationOutMax=[]  PParamMin=[]  PParamMax=[]  IParamMin=[]  IParamMax=[]  DParamMin=[]  DParamMax=[]  NParamMin=[]  NParamMax=[]  KbParamMin=[]  KbParamMax=[]  KtParamMin=[]  KtParamMax=[]  KbOutMin=[]  KbOutMax=[]  KtOutMin=[]  KtOutMax=[]  IntegratorOutMin=[]  IntegratorOutMax=[]  FilterOutMin=[]  FilterOutMax=[]  SumI1OutMin=[]  SumI1OutMax=[]  SumI2OutMin=[]  SumI2OutMax=[]  SumI3OutMin=[]  SumI3OutMax=[]  SumI4OutMin=[]  SumI4OutMax=[]  SumDOutMin=[]  SumDOutMax=[]  DifferentiatorOutMin=[]  DifferentiatorOutMax=[]  FilterDiffOutCoefMin=[]  FilterDiffOutCoefMax=[]  ReciprocalOutMin=[]  ReciprocalOutMax=[]  SumDenOutMin=[]  SumDenOutMax=[]  SumNumOutMin=[]  SumNumOutMax=[]  DivideOutMin=[]  DivideOutMax=[]  UdiffTsProdOutMin=[]  UdiffTsProdOutMax=[]  NTsProdOutMin=[]  NTsProdOutMax=[]  UintegralTsProdOutMin=[]  UintegralTsProdOutMax=[]  UngainTsProdOutMin=[]  UngainTsProdOutMax=[]  ClampingZeroOutDataTypeStr=Inherit: Inherit via back propagation  ClampingZeroOutMin=[]  ClampingZeroOutMax=[]  FilterDenConstantOutDataTypeStr=Inherit: Inherit via back propagation  FilterDenConstantOutMin=[]  FilterDenConstantOutMax=[]  PCopyOutDataTypeStr=Inherit: Inherit via back propagation  PCopyOutMin=[]  PCopyOutMax=[]  NCopyOutDataTypeStr=Inherit: Inherit via back propagation  NCopyOutMin=[]  NCopyOutMax=[]  IntegratorContinuousStateAttributes=''  IntegratorStateMustResolveToSignalObject=off  IntegratorRTWStateStorageClass=Auto  FilterContinuousStateAttributes=''  FilterStateMustResolveToSignalObject=off  FilterRTWStateStorageClass=Auto  ParallelPVariant=InternalParameters  IdealPVariant=Disabled  IVariant=InternalParameters  DVariant=Disabled  IntegratorVariant=Discrete  SatVariant=Disabled  AWVariant=Passthrough  PCopyVariant=Disabled  TRVariant=Disabled  FdbkBlocksVariant=Forward  IdealPFdbkVariant=Disabled  SatFdbkVariant=Disabled  DerivativeFilterVariant=Disabled  NVariant=Disabled  NCopyVariant=Disabled_SignalSpec  FilterICVariant=Disabled  IntegratorICVariant=InternalICs  ExternalResetVariant=Disabled  TRSumVariant=Passthrough  SumFdbkVariant=Disabled  SumVariant=Sum_PI  TsampFilterVariant=InternalTs  TsampNgainVariant=Passthrough  TsampIntegralVariant=Passthrough  ExternalSaturationOutDataTypeStr=Inherit: Same as second input
  Scope1 : Scope
  Scope2 : Scope
  Scope4 : Scope  NumInputPorts=2
  Sqrt : Sqrt
  Trigonometric Function : Trigonometry  Operator=cos
  Trigonometric Function1 : Trigonometry
  theta : Outport
  wires:
  alpha/1 -> Divide1/1, Math Function/1
  beta/1 -> Divide/1, Math Function1/1
  Math Function1/1 -> Add/2
  Math Function/1 -> Add/1
  Add/1 -> Sqrt/1
  Divide1/1 -> Scope4/1, Divide2/1
  Divide/1 -> Scope4/2, Divide3/1
  Divide2/1 -> Add1/1
  Divide3/1 -> Add1/2
  Add1/1 -> Scope1/1, PID Controller/1
  PID Controller/1 -> Discrete-Time Integrator/1
  Discrete-Time Integrator/1 -> Mod/1, Trigonometric Function/1, Trigonometric Function1/1  "theta"
  Trigonometric Function1/1 -> Divide2/2
  Trigonometric Function/1 -> Divide3/2
  Sqrt/1 -> Divide1/2, Divide/2
  Constant/1 -> Mod/2
  Mod/1 -> Scope2/1, theta/1

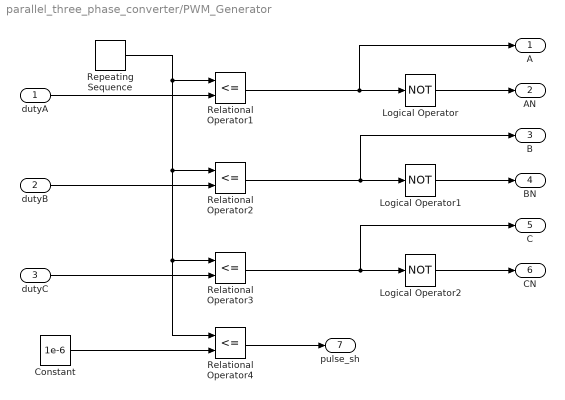
== system parallel_three_phase_converter/PWM_Generator ==
  dutyA : Inport
  dutyB : Inport  Port=2
  dutyC : Inport  Port=3
  Constant : Constant  Value=1e-6
  Logical Operator : Logic  Operator=NOT  AllPortsSameDT=off  OutDataTypeStr=boolean
  Logical Operator1 : Logic  Operator=NOT  AllPortsSameDT=off  OutDataTypeStr=boolean
  Logical Operator2 : Logic  Operator=NOT  AllPortsSameDT=off  OutDataTypeStr=boolean
  Relational Operator{1..4} (4 alike) : RelationalOperator  Operator=<=  OutDataTypeStr=boolean  RndMeth=Simplest  InputSameDT=off
  Repeating Sequence : simulink/Sources/Repeating Sequence  rep_seq_t=[0 0.25e-4 0.5e-4]  rep_seq_y=[0 1 0]
  A : Outport
  AN : Outport  Port=2
  B : Outport  Port=3
  BN : Outport  Port=4
  C : Outport  Port=5
  CN : Outport  Port=6
  pulse_sh : Outport  Port=7
  wires:
  Logical Operator/1 -> AN/1
  Logical Operator1/1 -> BN/1
  Relational Operator1/1 -> A/1, Logical Operator/1
  Relational Operator3/1 -> C/1, Logical Operator2/1
  Relational Operator2/1 -> B/1, Logical Operator1/1
  Repeating Sequence/1 -> Relational Operator4/1, Relational Operator3/1, Relational Operator2/1, Relational Operator1/1
  dutyC/1 -> Relational Operator3/2
  dutyB/1 -> Relational Operator2/2
  Logical Operator2/1 -> CN/1
  dutyA/1 -> Relational Operator1/2
  Constant/1 -> Relational Operator4/2
  Relational Operator4/1 -> pulse_sh/1

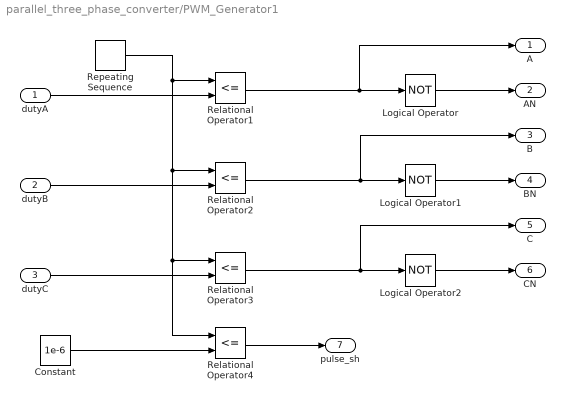
== system parallel_three_phase_converter/PWM_Generator1 ==
  dutyA : Inport
  dutyB : Inport  Port=2
  dutyC : Inport  Port=3
  Constant : Constant  Value=1e-6
  Logical Operator : Logic  Operator=NOT  AllPortsSameDT=off  OutDataTypeStr=boolean
  Logical Operator1 : Logic  Operator=NOT  AllPortsSameDT=off  OutDataTypeStr=boolean
  Logical Operator2 : Logic  Operator=NOT  AllPortsSameDT=off  OutDataTypeStr=boolean
  Relational Operator{1..4} (4 alike) : RelationalOperator  Operator=<=  OutDataTypeStr=boolean  RndMeth=Simplest  InputSameDT=off
  Repeating Sequence : simulink/Sources/Repeating Sequence  rep_seq_t=[0 0.25e-4 0.5e-4]  rep_seq_y=[0 1 0]
  A : Outport
  AN : Outport  Port=2
  B : Outport  Port=3
  BN : Outport  Port=4
  C : Outport  Port=5
  CN : Outport  Port=6
  pulse_sh : Outport  Port=7
  wires:
  Logical Operator/1 -> AN/1
  Logical Operator1/1 -> BN/1
  Relational Operator1/1 -> A/1, Logical Operator/1
  Relational Operator3/1 -> C/1, Logical Operator2/1
  Relational Operator2/1 -> B/1, Logical Operator1/1
  Repeating Sequence/1 -> Relational Operator4/1, Relational Operator3/1, Relational Operator2/1, Relational Operator1/1
  dutyC/1 -> Relational Operator3/2
  dutyB/1 -> Relational Operator2/2
  Logical Operator2/1 -> CN/1
  dutyA/1 -> Relational Operator1/2
  Constant/1 -> Relational Operator4/2
  Relational Operator4/1 -> pulse_sh/1

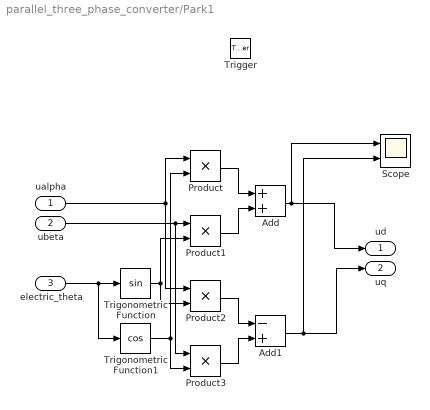
== system parallel_three_phase_converter/Park1 ==
  ualpha : Inport
  ubeta : Inport  Port=2
  electric_theta : Inport  Port=3
  Trigger : TriggerPort  VariantControl=(inherit)
  Add : Sum
  Add1 : Sum  Inputs=-+
  Product{,1..3} (4 alike) : Product
  Scope : Scope  NumInputPorts=2
  Trigonometric Function : Trigonometry
  Trigonometric Function1 : Trigonometry  Operator=cos
  ud : Outport
  uq : Outport  Port=2
  wires:
  electric_theta/1 -> Trigonometric Function1/1, Trigonometric Function/1
  Trigonometric Function1/1 -> Product3/2, Product/2
  ubeta/1 -> Product3/1, Product1/1
  Trigonometric Function/1 -> Product2/2, Product1/2
  Product/1 -> Add/1
  Product1/1 -> Add/2
  Product2/1 -> Add1/1
  Product3/1 -> Add1/2
  Add/1 -> ud/1, Scope/1
  Add1/1 -> uq/1, Scope/2
  ualpha/1 -> Product/1, Product2/1

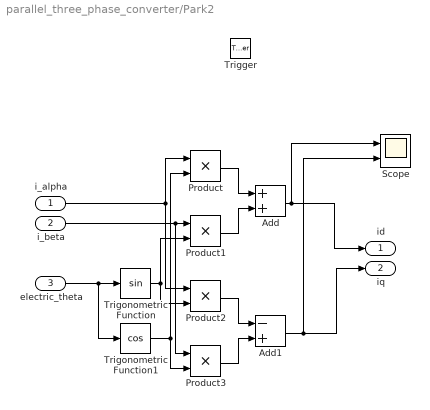
== system parallel_three_phase_converter/Park2 ==
  i_alpha : Inport
  i_beta : Inport  Port=2
  electric_theta : Inport  Port=3
  Trigger : TriggerPort  VariantControl=(inherit)
  Add : Sum
  Add1 : Sum  Inputs=-+
  Product{,1..3} (4 alike) : Product
  Scope : Scope  NumInputPorts=2
  Trigonometric Function : Trigonometry
  Trigonometric Function1 : Trigonometry  Operator=cos
  id : Outport
  iq : Outport  Port=2
  wires:
  electric_theta/1 -> Trigonometric Function1/1, Trigonometric Function/1
  Trigonometric Function1/1 -> Product3/2, Product/2
  i_beta/1 -> Product3/1, Product1/1
  Trigonometric Function/1 -> Product2/2, Product1/2
  Product/1 -> Add/1
  Product1/1 -> Add/2
  Product2/1 -> Add1/1
  Product3/1 -> Add1/2
  Add/1 -> id/1, Scope/1
  Add1/1 -> iq/1, Scope/2
  i_alpha/1 -> Product/1, Product2/1

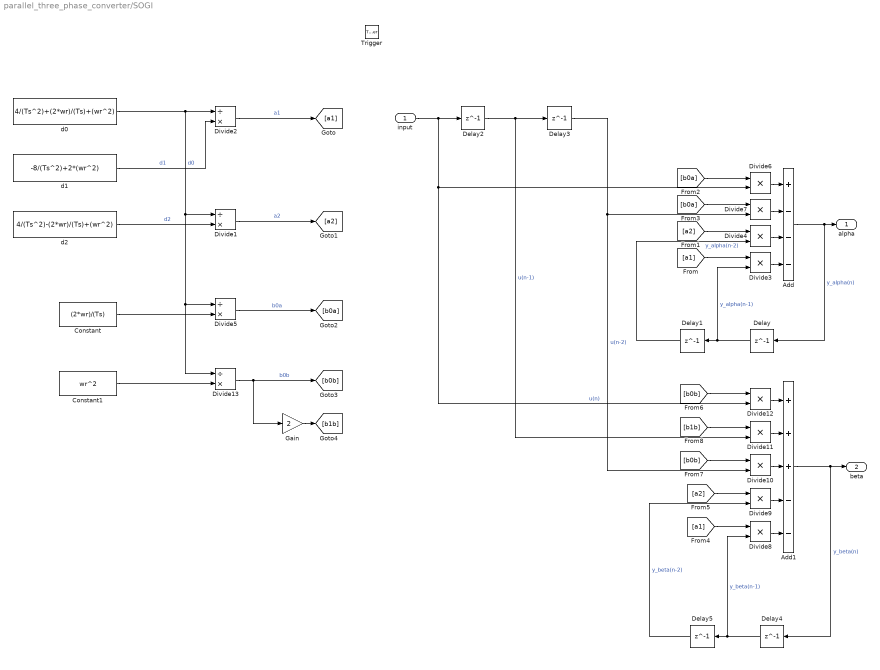
== system parallel_three_phase_converter/SOGI ==
  input : Inport
  Trigger : TriggerPort  VariantControl=(inherit)
  Add : Sum  Inputs=+---
  Add1 : Sum  Inputs=+++--
  Constant : Constant  Value=(2*wr)/(Ts)
  Constant1 : Constant  Value=wr^2
  Delay{,1..5} (6 alike) : Delay  DelayLength=1  InitialCondition=0
  Divide{1..2,5,13} (4 alike) : Product  Inputs=/*
  Divide{3..4,6..12} (9 alike) : Product  Inputs=**
  Gain : Gain  Gain=2
  d0 : Constant  Value=4/(Ts^2)+(2*wr)/(Ts)+(wr^2)
  d1 : Constant  Value=-8/(Ts^2)+2*(wr^2)
  d2 : Constant  Value=4/(Ts^2)-(2*wr)/(Ts)+(wr^2)
  alpha : Outport
  beta : Outport  Port=2
  wires:
  d0/1 -> Divide2/1, Divide5/1, Divide13/1, Divide1/1  "d0"
  d1/1 -> Divide2/2  "d1"
  d2/1 -> Divide1/2  "d2"
  Divide2/1 -> [a1]  "a1"
  Divide1/1 -> [a2]  "a2"
  Add/1 -> Delay/1, alpha/1  "y_alpha(n)"
  Delay/1 -> Divide3/2, Delay1/1  "y_alpha(n-1)"
  Delay1/1 -> Divide4/2  "y_alpha(n-2)"
  Divide3/1 -> Add/4
  [a1] -> Divide3/1
  Divide4/1 -> Add/3
  [a2] -> Divide4/1
  Divide5/1 -> [b0a]  "b0a"
  Constant/1 -> Divide5/2
  Divide6/1 -> Add/1
  [b0a] -> Divide6/1
  Divide7/1 -> Add/2
  input/1 -> Divide12/2, Divide6/2, Delay2/1  "u(n)"
  Delay2/1 -> Divide11/2, Delay3/1  "u(n-1)"
  Delay3/1 -> Divide10/2, Divide7/2  "u(n-2)"
  [b0a] -> Divide7/1
  Add1/1 -> Delay4/1, beta/1  "y_beta(n)"
  Delay5/1 -> Divide9/2  "y_beta(n-2)"
  Delay4/1 -> Divide8/2, Delay5/1  "y_beta(n-1)"
  Divide8/1 -> Add1/5
  [a1] -> Divide8/1
  Divide9/1 -> Add1/4
  [a2] -> Divide9/1
  Divide10/1 -> Add1/3
  Divide11/1 -> Add1/2
  Divide12/1 -> Add1/1
  Constant1/1 -> Divide13/2
  Divide13/1 -> Gain/1, [b0b]  "b0b"
  Gain/1 -> [b1b]
  [b0b] -> Divide12/1
  [b0b] -> Divide10/1
  [b1b] -> Divide11/1

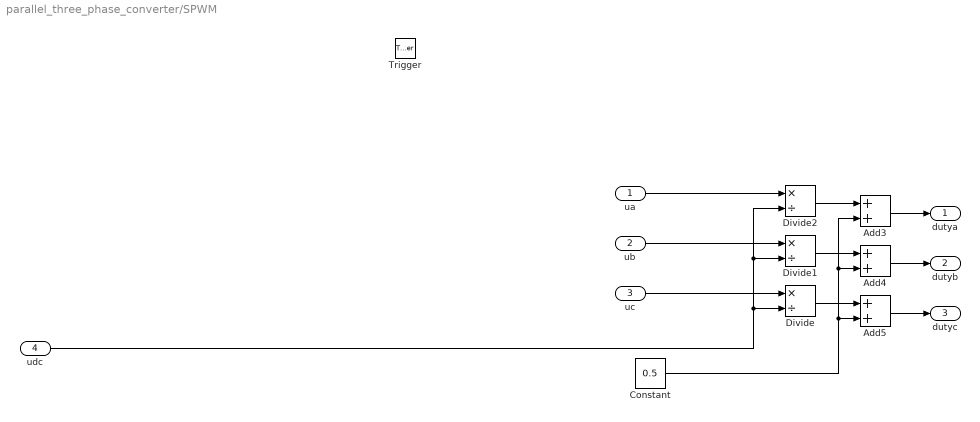
== system parallel_three_phase_converter/SPWM ==
  ua : Inport
  ub : Inport  Port=2
  uc : Inport  Port=3
  udc : Inport  Port=4
  Trigger : TriggerPort  VariantControl=(inherit)
  Add3 : Sum
  Add4 : Sum
  Add5 : Sum
  Constant : Constant  Value=0.5
  Divide : Product  Inputs=*/
  Divide1 : Product  Inputs=*/
  Divide2 : Product  Inputs=*/
  dutya : Outport
  dutyb : Outport  Port=2
  dutyc : Outport  Port=3
  wires:
  udc/1 -> Divide/2, Divide2/2, Divide1/2
  ua/1 -> Divide2/1
  uc/1 -> Divide/1
  Divide2/1 -> Add3/1
  Divide1/1 -> Add4/1
  Divide/1 -> Add5/1
  Constant/1 -> Add5/2, Add4/2, Add3/2
  Add3/1 -> dutya/1
  Add4/1 -> dutyb/1
  Add5/1 -> dutyc/1
  ub/1 -> Divide1/1

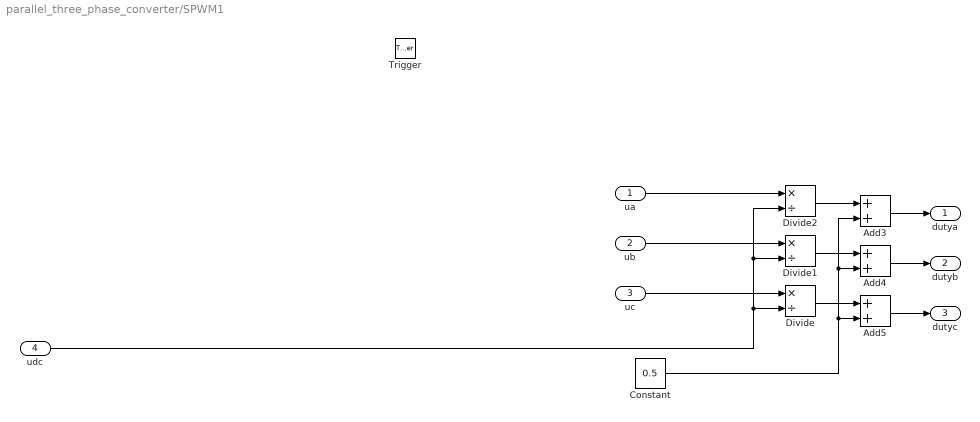
== system parallel_three_phase_converter/SPWM1 ==
  ua : Inport
  ub : Inport  Port=2
  uc : Inport  Port=3
  udc : Inport  Port=4
  Trigger : TriggerPort  VariantControl=(inherit)
  Add3 : Sum
  Add4 : Sum
  Add5 : Sum
  Constant : Constant  Value=0.5
  Divide : Product  Inputs=*/
  Divide1 : Product  Inputs=*/
  Divide2 : Product  Inputs=*/
  dutya : Outport
  dutyb : Outport  Port=2
  dutyc : Outport  Port=3
  wires:
  udc/1 -> Divide/2, Divide2/2, Divide1/2
  ua/1 -> Divide2/1
  uc/1 -> Divide/1
  Divide2/1 -> Add3/1
  Divide1/1 -> Add4/1
  Divide/1 -> Add5/1
  Constant/1 -> Add5/2, Add4/2, Add3/2
  Add3/1 -> dutya/1
  Add4/1 -> dutyb/1
  Add5/1 -> dutyc/1
  ub/1 -> Divide1/1
